simulink model "Test_openloop"  (R2017b)
settings: Solver=ode45  StartTime=0.0  StopTime=10  RelTol=1e-3
values from neighbouring files (symbols this model uses):
  Cdv = 0.02    [params.m]
  D = 0.55    [params.m]
  Ix = 1    [params.m]
  Ixy = 0.2    [params.m]
  Iy = 1    [params.m]
  Iz = 1    [params.m]
  Lx = b/2 + L_kr / sqrt(1 + tan(phi_kr1)^2 + tan(phi_kr1)^2)    [params.m]
  Ly = L_kr / sqrt(1 + tan(phi_kr1)^2 + tan(phi_kr1)^2) * tan(phi_kr2)    [params.m]
  Lz = a/2 + L_kr / sqrt(1 + tan(phi_kr1)^2 + tan(phi_kr1)^2) * tan(phi_kr1)    [params.m]
  M = [m 0 0 0 0 0 ... (first row only)    [params.m]
  m = 1    [params.m]
  rho = 1.22    [params.m]
  x_c = 0    [params.m]
  y_c = 0.005    [params.m]
settings Model: Creator=alexeimargun  LastModifiedBy=alexeimargun
settings DataIOCC: SaveFormat=StructureWithTime
settings OptimizationCC: LifeSpan=inf
settings DebuggingCC: SFExecutionAtInitializationDiag=none
settings HardwareCC: ProdBitPerSizeT=32  ProdBitPerPtrDiffT=32  ProdWordSize=32  ProdHWDeviceType=Specified
settings CodeAppCC: StateflowObjectComments=on
settings GRTTargetCC: GeneratePreprocessorConditionals=Disable all

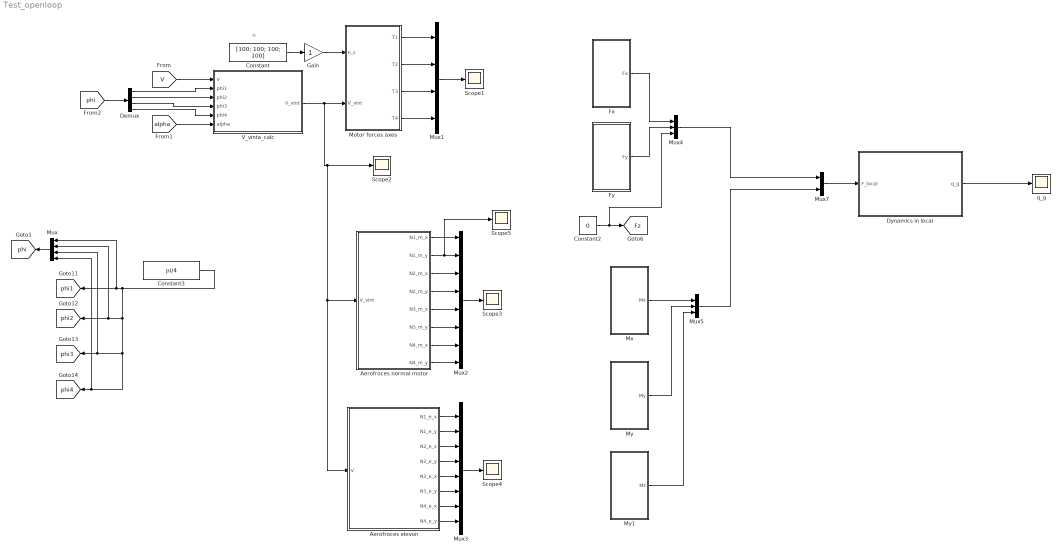
== system Test_openloop ==
  note: n
  Aerofroces elevon : Subsystem
  Aerofroces normal motor : Subsystem
  Constant : Constant  Value=[100; 100; 100; 100]
  Constant2 : Constant  Value=0
  Constant3 : Constant  Value=pi/4
  Demux : Demux
  Dynamics in local : Subsystem
  Fx : Subsystem
  Fy : Subsystem
  Gain : Gain
  Motor forces axes : Subsystem
  Mux : Mux
  Mux1 : Mux
  Mux2 : Mux  Inputs=8
  Mux3 : Mux  Inputs=8
  Mux4 : Mux  Inputs=3
  Mux5 : Mux  Inputs=3
  Mux7 : Mux  Inputs=2
  Mx : Subsystem
  My : Subsystem
  My1 : Subsystem
  Scope{1..5} (5 alike) : Scope
  V_vinta_calc : MATLAB Function  TreatAsAtomicUnit=on
  q_g : Scope
  tag scope: Fz=global, phi1=global, phi2=global, phi3=global, phi4=global, phi=global
  wires:
  Dynamics in local/1(q_g) -> q_g/1
  Motor forces axes/2(T2) -> Mux1/2
  Mux1/1 -> Scope1/1
  Motor forces axes/1(T1) -> Mux1/1
  Constant/1 -> Gain/1
  Motor forces axes/3(T3) -> Mux1/3
  Motor forces axes/4(T4) -> Mux1/4
  [V] -> V_vinta_calc/1(V)
  [alpha] -> V_vinta_calc/6(alpha)
  Gain/1 -> Motor forces axes/1(n_s)
  V_vinta_calc/1(V_vint) -> Aerofroces elevon/1(V), Aerofroces normal motor/1(V_vint), Scope2/1, Motor forces axes/2(V_vint)
  Aerofroces elevon/7(N4_e_x) -> Mux3/7
  Aerofroces elevon/3(N2_e_x) -> Mux3/3
  Aerofroces normal motor/4(N2_m_y) -> Mux2/4
  Aerofroces normal motor/7(N4_m_x) -> Mux2/7
  Aerofroces normal motor/5(N3_m_x) -> Mux2/5
  Aerofroces elevon/2(N1_e_y) -> Mux3/2
  Mux3/1 -> Scope4/1
  Aerofroces elevon/5(N3_e_x) -> Mux3/5
  Aerofroces normal motor/8(N4_m_y) -> Mux2/8
  Mux2/1 -> Scope3/1
  Aerofroces elevon/1(N1_e_x) -> Mux3/1
  Aerofroces normal motor/3(N2_m_x) -> Mux2/3
  Aerofroces elevon/6(N3_e_y) -> Mux3/6
  Aerofroces normal motor/6(N3_m_y) -> Mux2/6
  Aerofroces elevon/4(N2_e_y) -> Mux3/4
  Aerofroces elevon/8(N4_e_y) -> Mux3/8
  Aerofroces normal motor/2(N1_m_y) -> Scope5/1, Mux2/2
  Aerofroces normal motor/1(N1_m_x) -> Mux2/1
  Constant3/1 -> Mux/4, [phi4], Mux/3, [phi3], [phi2], Mux/2, [phi1], Mux/1
  Mux/1 -> [phi]
  [phi] -> Demux/1
  Demux/1 -> V_vinta_calc/2(phi1)
  Demux/2 -> V_vinta_calc/3(phi2)
  Demux/3 -> V_vinta_calc/4(phi3)
  Demux/4 -> V_vinta_calc/5(phi4)
  Constant2/1 -> Mux4/3, [Fz]
  Fy/1(Fy) -> Mux4/2
  Mux4/1 -> Mux7/1
  Mx/1(Mx) -> Mux5/1
  My/1(My) -> Mux5/2
  My1/1(Mz) -> Mux5/3
  Mux5/1 -> Mux7/2
  Fx/1(Fx) -> Mux4/1
  Mux7/1 -> Dynamics in local/1(F_local)

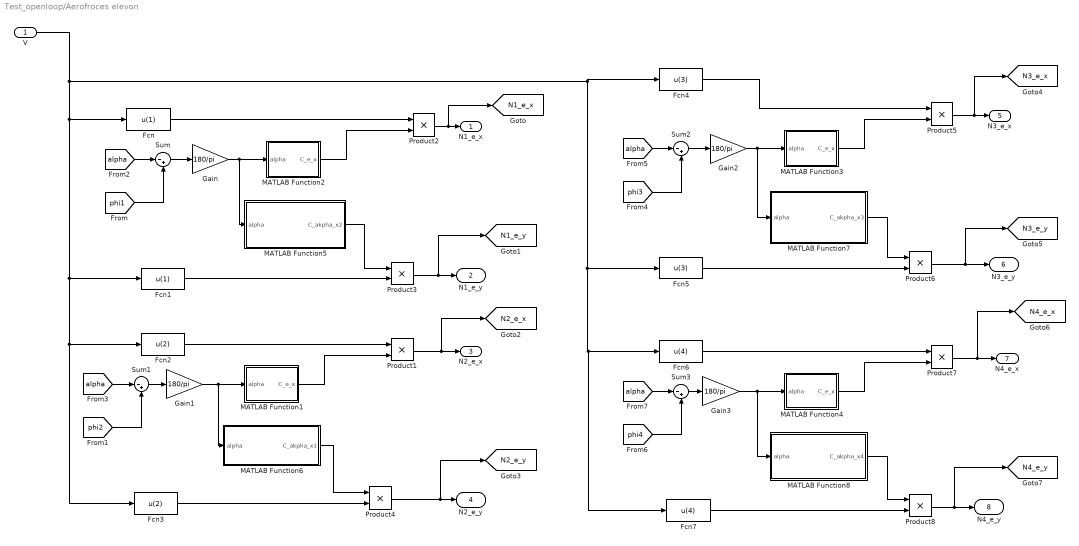
== system Test_openloop/Aerofroces elevon ==
  V : Inport
  Fcn : Fcn  Expr=u(1)
  Fcn1 : Fcn  Expr=u(1)
  Fcn2 : Fcn  Expr=u(2)
  Fcn3 : Fcn  Expr=u(2)
  Fcn4 : Fcn  Expr=u(3)
  Fcn5 : Fcn  Expr=u(3)
  Fcn6 : Fcn  Expr=u(4)
  Fcn7 : Fcn  Expr=u(4)
  Gain{,1..3} (4 alike) : Gain  Gain=180/pi
  MATLAB Function1 : MATLAB Function  TreatAsAtomicUnit=on
  MATLAB Function2 : MATLAB Function  TreatAsAtomicUnit=on
  MATLAB Function3 : MATLAB Function  TreatAsAtomicUnit=on
  MATLAB Function4 : MATLAB Function  TreatAsAtomicUnit=on
  MATLAB Function5 : MATLAB Function  TreatAsAtomicUnit=on
  MATLAB Function6 : MATLAB Function  TreatAsAtomicUnit=on
  MATLAB Function7 : MATLAB Function  TreatAsAtomicUnit=on
  MATLAB Function8 : MATLAB Function  TreatAsAtomicUnit=on
  Product{1..8} (8 alike) : Product
  Sum{,1..3} (4 alike) : Sum  Inputs=|-+
  N1_e_x : Outport
  N1_e_y : Outport  Port=2
  N2_e_x : Outport  Port=3
  N2_e_y : Outport  Port=4
  N3_e_x : Outport  Port=5
  N3_e_y : Outport  Port=6
  N4_e_x : Outport  Port=7
  N4_e_y : Outport  Port=8
  tag scope: N1_e_x=global, N1_e_y=global, N2_e_x=global, N2_e_y=global, N3_e_x=global, N3_e_y=global, N4_e_x=global, N4_e_y=global
  wires:
  Product3/1 -> [N1_e_y], N1_e_y/1
  Product2/1 -> [N1_e_x], N1_e_x/1
  Sum/1 -> Gain/1
  MATLAB Function5/1(C_akpha_x2) -> Product3/1
  MATLAB Function2/1(C_e_x) -> Product2/2
  [alpha] -> Sum1/1
  [phi2] -> Sum1/2
  V/1 -> Fcn7/1, Fcn6/1, Fcn5/1, Fcn4/1, Fcn2/1, Fcn3/1, Fcn1/1, Fcn/1
  MATLAB Function1/1(C_e_x) -> Product1/2
  MATLAB Function6/1(C_akpha_x1) -> Product4/1
  Sum1/1 -> Gain1/1
  Product1/1 -> [N2_e_x], N2_e_x/1
  Product4/1 -> [N2_e_y], N2_e_y/1
  Product6/1 -> [N3_e_y], N3_e_y/1
  Product5/1 -> [N3_e_x], N3_e_x/1
  Sum2/1 -> Gain2/1
  MATLAB Function7/1(C_akpha_x3) -> Product6/1
  MATLAB Function3/1(C_e_x) -> Product5/2
  [phi3] -> Sum2/2
  [alpha] -> Sum2/1
  [alpha] -> Sum3/1
  [phi4] -> Sum3/2
  MATLAB Function4/1(C_e_x) -> Product7/2
  MATLAB Function8/1(C_akpha_x4) -> Product8/1
  Sum3/1 -> Gain3/1
  Product7/1 -> [N4_e_x], N4_e_x/1
  Product8/1 -> [N4_e_y], N4_e_y/1
  Gain/1 -> MATLAB Function5/1(alpha), MATLAB Function2/1(alpha)
  Gain1/1 -> MATLAB Function6/1(alpha), MATLAB Function1/1(alpha)
  Gain2/1 -> MATLAB Function7/1(alpha), MATLAB Function3/1(alpha)
  Gain3/1 -> MATLAB Function8/1(alpha), MATLAB Function4/1(alpha)
  Fcn/1 -> Product2/1
  Fcn1/1 -> Product3/2
  Fcn2/1 -> Product1/1
  Fcn3/1 -> Product4/2
  Fcn4/1 -> Product5/1
  Fcn5/1 -> Product6/2
  Fcn6/1 -> Product7/1
  Fcn7/1 -> Product8/2
  [alpha] -> Sum/1
  [phi1] -> Sum/2

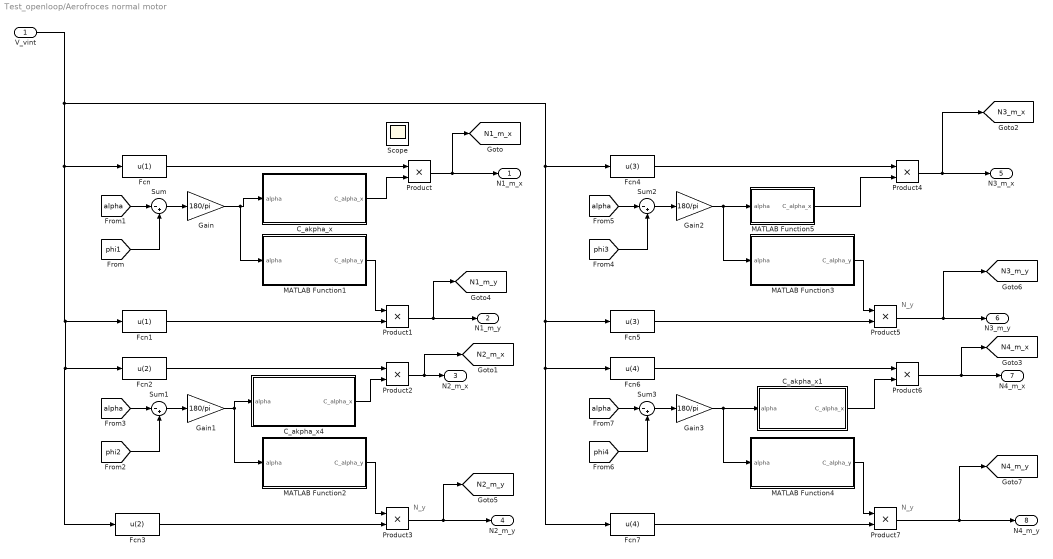
== system Test_openloop/Aerofroces normal motor ==
  note: N_y
  note: N_y
  note: N_y
  V_vint : Inport
  C_akpha_x : MATLAB Function  TreatAsAtomicUnit=on
  C_akpha_x1 : MATLAB Function  TreatAsAtomicUnit=on
  C_akpha_x4 : MATLAB Function  TreatAsAtomicUnit=on
  Fcn : Fcn  Expr=u(1)
  Fcn1 : Fcn  Expr=u(1)
  Fcn2 : Fcn  Expr=u(2)
  Fcn3 : Fcn  Expr=u(2)
  Fcn4 : Fcn  Expr=u(3)
  Fcn5 : Fcn  Expr=u(3)
  Fcn6 : Fcn  Expr=u(4)
  Fcn7 : Fcn  Expr=u(4)
  Gain{,1..3} (4 alike) : Gain  Gain=180/pi
  MATLAB Function1 : MATLAB Function  TreatAsAtomicUnit=on
  MATLAB Function2 : MATLAB Function  TreatAsAtomicUnit=on
  MATLAB Function3 : MATLAB Function  TreatAsAtomicUnit=on
  MATLAB Function4 : MATLAB Function  TreatAsAtomicUnit=on
  MATLAB Function5 : MATLAB Function  TreatAsAtomicUnit=on
  Product{,1..7} (8 alike) : Product
  Scope : Scope
  Sum{,1..3} (4 alike) : Sum  Inputs=|-+
  N1_m_x : Outport
  N1_m_y : Outport  Port=2
  N2_m_x : Outport  Port=3
  N2_m_y : Outport  Port=4
  N3_m_x : Outport  Port=5
  N3_m_y : Outport  Port=6
  N4_m_x : Outport  Port=7
  N4_m_y : Outport  Port=8
  tag scope: N1_m_x=global, N1_m_y=global, N2_m_x=global, N2_m_y=global, N3_m_x=global, N3_m_y=global, N4_m_x=global, N4_m_y=global
  wires:
  Product1/1 -> [N1_m_y], N1_m_y/1
  C_akpha_x/1(C_alpha_x) -> Product/2
  MATLAB Function1/1(C_alpha_y) -> Product1/1
  [alpha] -> Sum/1
  Sum/1 -> Gain/1
  [phi1] -> Sum/2
  Gain1/1 -> MATLAB Function2/1(alpha), C_akpha_x4/1(alpha)
  [phi2] -> Sum1/2
  Sum1/1 -> Gain1/1
  [alpha] -> Sum1/1
  MATLAB Function2/1(C_alpha_y) -> Product3/1
  C_akpha_x4/1(C_alpha_x) -> Product2/2
  Product2/1 -> [N2_m_x], N2_m_x/1
  Product3/1 -> [N2_m_y], N2_m_y/1
  Product7/1 -> [N4_m_y], N4_m_y/1
  Product6/1 -> [N4_m_x], N4_m_x/1
  V_vint/1 -> Fcn5/1, Fcn6/1, Fcn7/1, Fcn4/1, Fcn/1, Fcn3/1, Fcn2/1, Fcn1/1
  C_akpha_x1/1(C_alpha_x) -> Product6/2
  MATLAB Function4/1(C_alpha_y) -> Product7/1
  [alpha] -> Sum3/1
  Sum3/1 -> Gain3/1
  [phi4] -> Sum3/2
  Gain3/1 -> MATLAB Function4/1(alpha), C_akpha_x1/1(alpha)
  Gain2/1 -> MATLAB Function3/1(alpha), MATLAB Function5/1(alpha)
  [phi3] -> Sum2/2
  Sum2/1 -> Gain2/1
  [alpha] -> Sum2/1
  MATLAB Function3/1(C_alpha_y) -> Product5/1
  MATLAB Function5/1(C_alpha_x) -> Product4/2
  Product4/1 -> [N3_m_x], N3_m_x/1
  Product5/1 -> [N3_m_y], N3_m_y/1
  Product/1 -> [N1_m_x], N1_m_x/1
  Gain/1 -> MATLAB Function1/1(alpha), C_akpha_x/1(alpha)
  Fcn/1 -> Product/1
  Fcn1/1 -> Product1/2
  Fcn2/1 -> Product2/1
  Fcn3/1 -> Product3/2
  Fcn4/1 -> Product4/1
  Fcn5/1 -> Product5/2
  Fcn6/1 -> Product6/1
  Fcn7/1 -> Product7/2

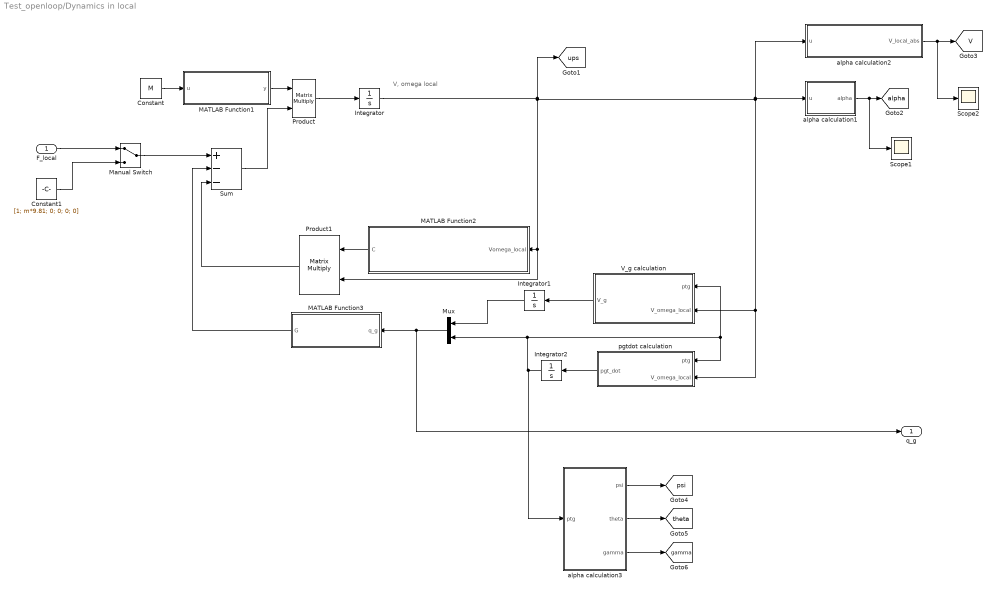
== system Test_openloop/Dynamics in local ==
  note: V, omega local
  F_local : Inport
  Constant : Constant  Value=M
  Constant1 : Constant  Value=[1; m*9.81; 0; 0; 0; 0]
  Integrator : Integrator
  Integrator1 : Integrator  InitialCondition=[0;0;0]
  Integrator2 : Integrator  InitialCondition=[0;0;0]
  MATLAB Function1 : MATLAB Function  TreatAsAtomicUnit=on
  MATLAB Function2 : MATLAB Function  TreatAsAtomicUnit=on
  MATLAB Function3 : MATLAB Function  TreatAsAtomicUnit=on
  Manual Switch : ManualSwitch
  Mux : Mux  Inputs=2
  Product : Product  Multiplication=Matrix(*)
  Product1 : Product  Multiplication=Matrix(*)
  Scope1 : Scope
  Scope2 : Scope
  Sum : Sum  Inputs=+--
  V_g calculation : MATLAB Function  TreatAsAtomicUnit=on
  alpha calculation1 : MATLAB Function  TreatAsAtomicUnit=on
  alpha calculation2 : MATLAB Function  TreatAsAtomicUnit=on
  alpha calculation3 : MATLAB Function  TreatAsAtomicUnit=on
  pgtdot calculation : MATLAB Function  TreatAsAtomicUnit=on
  q_g : Outport
  tag scope: V=global, alpha=global, gamma=global, psi=global, theta=global, ups=global
  wires:
  MATLAB Function1/1(y) -> Product/1
  Product1/1 -> Sum/3
  Integrator2/1 -> alpha calculation3/1(ptg), V_g calculation/1(ptg), pgtdot calculation/1(ptg), Mux/2
  Integrator/1 -> Product1/2, MATLAB Function2/1(Vomega_local), alpha calculation2/1(u), alpha calculation1/1(u), V_g calculation/2(V_omega_local), pgtdot calculation/2(V_omega_local), [ups]
  Mux/1 -> q_g/1, MATLAB Function3/1(q_g)
  pgtdot calculation/1(pgt_dot) -> Integrator2/1
  MATLAB Function3/1(G) -> Sum/2
  Sum/1 -> Product/2
  Integrator1/1 -> Mux/1
  Constant/1 -> MATLAB Function1/1(u)
  MATLAB Function2/1(C) -> Product1/1
  Product/1 -> Integrator/1
  V_g calculation/1(V_g) -> Integrator1/1
  alpha calculation1/1(alpha) -> Scope1/1, [alpha]
  alpha calculation2/1(V_local_abs) -> Scope2/1, [V]
  Constant1/1 -> Manual Switch/2
  Manual Switch/1 -> Sum/1
  F_local/1 -> Manual Switch/1
  alpha calculation3/1(psi) -> [psi]
  alpha calculation3/2(theta) -> [theta]
  alpha calculation3/3(gamma) -> [gamma]

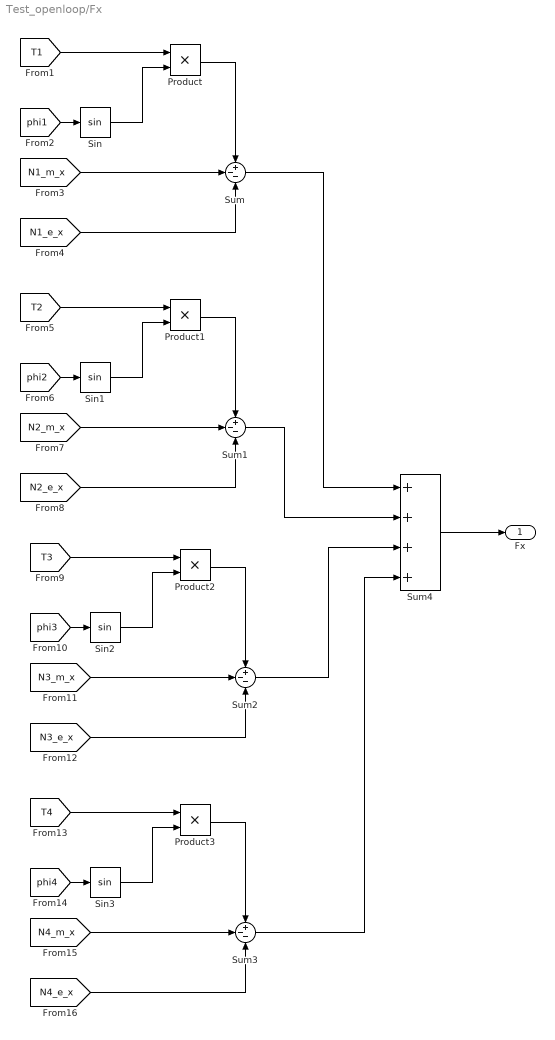
== system Test_openloop/Fx ==
  Product{,1..3} (4 alike) : Product
  Sin{,1..3} (4 alike) : Trigonometry
  Sum{,1..3} (4 alike) : Sum  Inputs=+--
  Sum4 : Sum  Inputs=++++
  Fx : Outport
  wires:
  [phi3] -> Sin2/1
  Product2/1 -> Sum2/1
  Sin2/1 -> Product2/2
  [phi4] -> Sin3/1
  [N3_e_x] -> Sum2/3
  [T1] -> Product/1
  Product/1 -> Sum/1
  [T2] -> Product1/1
  Sin1/1 -> Product1/2
  [N2_m_x] -> Sum1/2
  Product3/1 -> Sum3/1
  Sum/1 -> Sum4/1
  [phi2] -> Sin1/1
  [N1_m_x] -> Sum/2
  [N1_e_x] -> Sum/3
  [T3] -> Product2/1
  Sin3/1 -> Product3/2
  Sin/1 -> Product/2
  [N4_m_x] -> Sum3/2
  [N3_m_x] -> Sum2/2
  [phi1] -> Sin/1
  [T4] -> Product3/1
  Sum2/1 -> Sum4/3
  Sum1/1 -> Sum4/2
  [N4_e_x] -> Sum3/3
  Product1/1 -> Sum1/1
  Sum3/1 -> Sum4/4
  [N2_e_x] -> Sum1/3
  Sum4/1 -> Fx/1

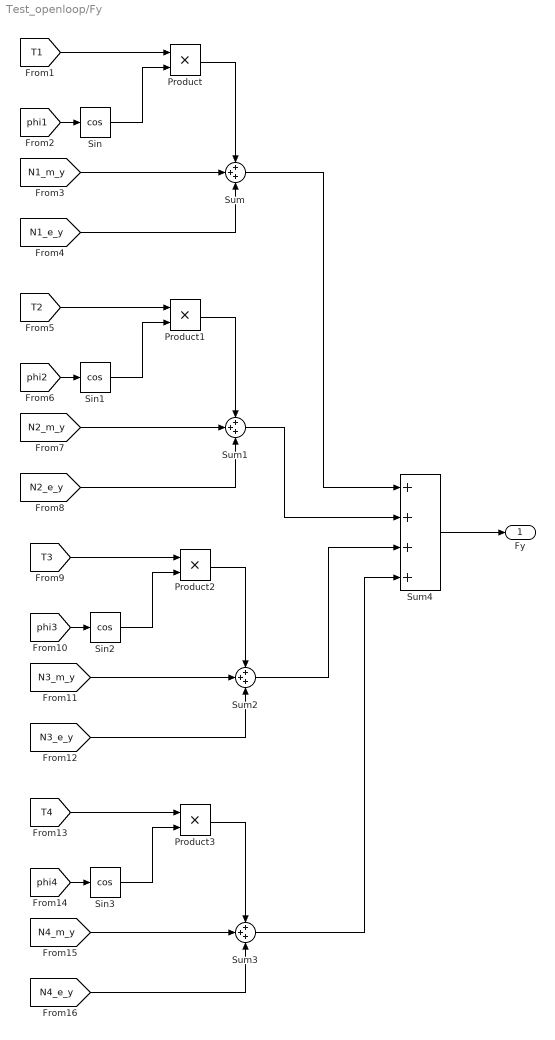
== system Test_openloop/Fy ==
  Product{,1..3} (4 alike) : Product
  Sin{,1..3} (4 alike) : Trigonometry  Operator=cos
  Sum{,1..3} (4 alike) : Sum  Inputs=+++
  Sum4 : Sum  Inputs=++++
  Fy : Outport
  wires:
  Sum4/1 -> Fy/1
  [N2_e_y] -> Sum1/3
  Sum3/1 -> Sum4/4
  Product1/1 -> Sum1/1
  [N4_e_y] -> Sum3/3
  Sum1/1 -> Sum4/2
  Sum2/1 -> Sum4/3
  [T4] -> Product3/1
  [phi1] -> Sin/1
  [N3_m_y] -> Sum2/2
  [N4_m_y] -> Sum3/2
  Sin/1 -> Product/2
  Sin3/1 -> Product3/2
  [T3] -> Product2/1
  [N1_e_y] -> Sum/3
  [N1_m_y] -> Sum/2
  [phi2] -> Sin1/1
  Sum/1 -> Sum4/1
  Product3/1 -> Sum3/1
  [N2_m_y] -> Sum1/2
  Sin1/1 -> Product1/2
  [T2] -> Product1/1
  Product/1 -> Sum/1
  [T1] -> Product/1
  [N3_e_y] -> Sum2/3
  [phi4] -> Sin3/1
  Sin2/1 -> Product2/2
  Product2/1 -> Sum2/1
  [phi3] -> Sin2/1

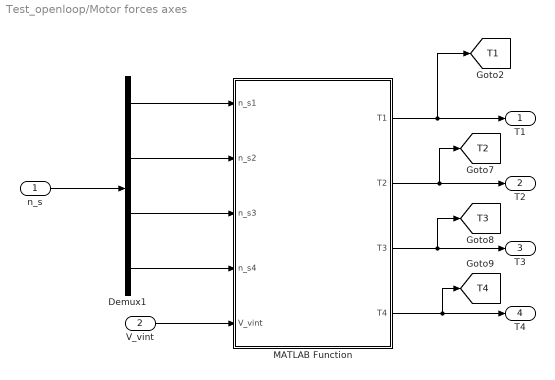
== system Test_openloop/Motor forces axes ==
  n_s : Inport
  V_vint : Inport  Port=2
  Demux1 : Demux
  MATLAB Function : MATLAB Function  TreatAsAtomicUnit=on
  T1 : Outport
  T2 : Outport  Port=2
  T3 : Outport  Port=3
  T4 : Outport  Port=4
  tag scope: T1=global, T2=global, T3=global, T4=global
  wires:
  MATLAB Function/3(T3) -> [T3], T3/1
  MATLAB Function/4(T4) -> [T4], T4/1
  Demux1/1 -> MATLAB Function/1(n_s1)
  Demux1/3 -> MATLAB Function/3(n_s3)
  Demux1/4 -> MATLAB Function/4(n_s4)
  V_vint/1 -> MATLAB Function/5(V_vint)
  MATLAB Function/2(T2) -> [T2], T2/1
  Demux1/2 -> MATLAB Function/2(n_s2)
  MATLAB Function/1(T1) -> [T1], T1/1
  n_s/1 -> Demux1/1

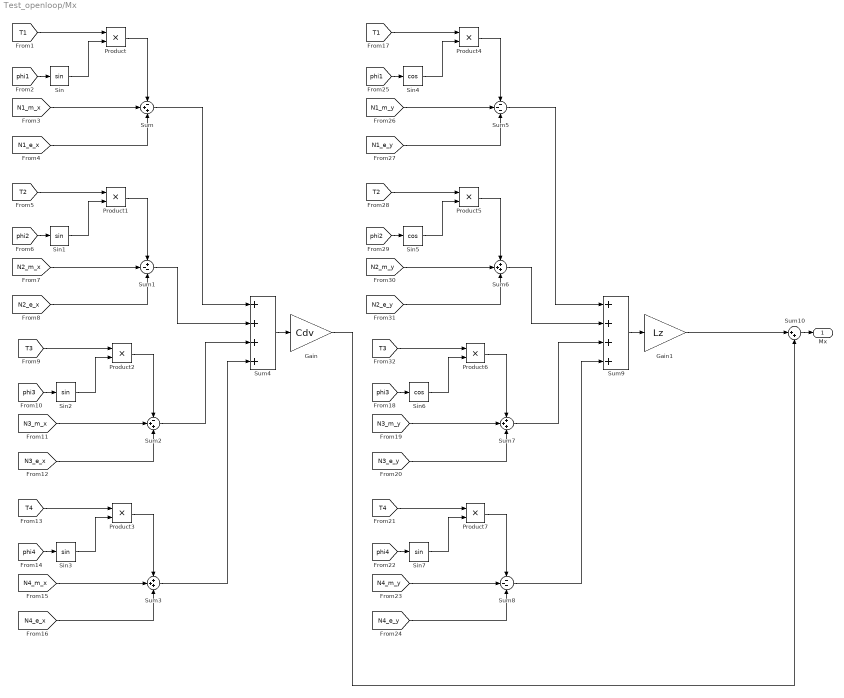
== system Test_openloop/Mx ==
  Gain : Gain  Gain=Cdv
  Gain1 : Gain  Gain=Lz
  Product{,1..7} (8 alike) : Product
  Sin{,1..3,7} (5 alike) : Trigonometry
  Sin4 : Trigonometry  Operator=cos
  Sin5 : Trigonometry  Operator=cos
  Sin6 : Trigonometry  Operator=cos
  Sum : Sum  Inputs=-++
  Sum1 : Sum  Inputs=+--
  Sum10 : Sum  Inputs=|++
  Sum2 : Sum  Inputs=-++
  Sum3 : Sum  Inputs=+++
  Sum4 : Sum  Inputs=++++
  Sum5 : Sum  Inputs=---
  Sum6 : Sum  Inputs=+++
  Sum7 : Sum  Inputs=+++
  Sum8 : Sum  Inputs=---
  Sum9 : Sum  Inputs=++++
  Mx : Outport
  wires:
  [N2_e_x] -> Sum1/3
  [phi3] -> Sin6/1
  Sum3/1 -> Sum4/4
  Product1/1 -> Sum1/1
  [N4_e_x] -> Sum3/3
  Sum8/1 -> Sum9/4
  Sum1/1 -> Sum4/2
  [N4_e_y] -> Sum8/3
  [T1] -> Product4/1
  Sin6/1 -> Product6/2
  Sum9/1 -> Gain1/1
  Product7/1 -> Sum8/1
  Sum5/1 -> Sum9/1
  Sum2/1 -> Sum4/3
  [T4] -> Product3/1
  [phi1] -> Sin/1
  Sum7/1 -> Sum9/3
  Product6/1 -> Sum7/1
  Sum6/1 -> Sum9/2
  [N3_e_y] -> Sum7/3
  [T3] -> Product6/1
  [N3_m_x] -> Sum2/2
  [phi1] -> Sin4/1
  [N4_m_x] -> Sum3/2
  Sin/1 -> Product/2
  Sin3/1 -> Product3/2
  Product4/1 -> Sum5/1
  [T3] -> Product2/1
  [phi2] -> Sin5/1
  Sin4/1 -> Product4/2
  Sum4/1 -> Gain/1
  [N1_e_x] -> Sum/3
  [N1_m_x] -> Sum/2
  [T2] -> Product5/1
  Sin7/1 -> Product7/2
  [phi2] -> Sin1/1
  [N1_e_y] -> Sum5/3
  Sum/1 -> Sum4/1
  [phi4] -> Sin7/1
  [T4] -> Product7/1
  Product3/1 -> Sum3/1
  Product5/1 -> Sum6/1
  [N2_m_x] -> Sum1/2
  Sin5/1 -> Product5/2
  Sin1/1 -> Product1/2
  Gain1/1 -> Sum10/1
  [N2_e_y] -> Sum6/3
  [N2_m_y] -> Sum6/2
  [N1_m_y] -> Sum5/2
  [T2] -> Product1/1
  Product/1 -> Sum/1
  [N3_m_y] -> Sum7/2
  [T1] -> Product/1
  [N3_e_x] -> Sum2/3
  [N4_m_y] -> Sum8/2
  Gain/1 -> Sum10/2
  Sum10/1 -> Mx/1
  [phi4] -> Sin3/1
  Sin2/1 -> Product2/2
  Product2/1 -> Sum2/1
  [phi3] -> Sin2/1

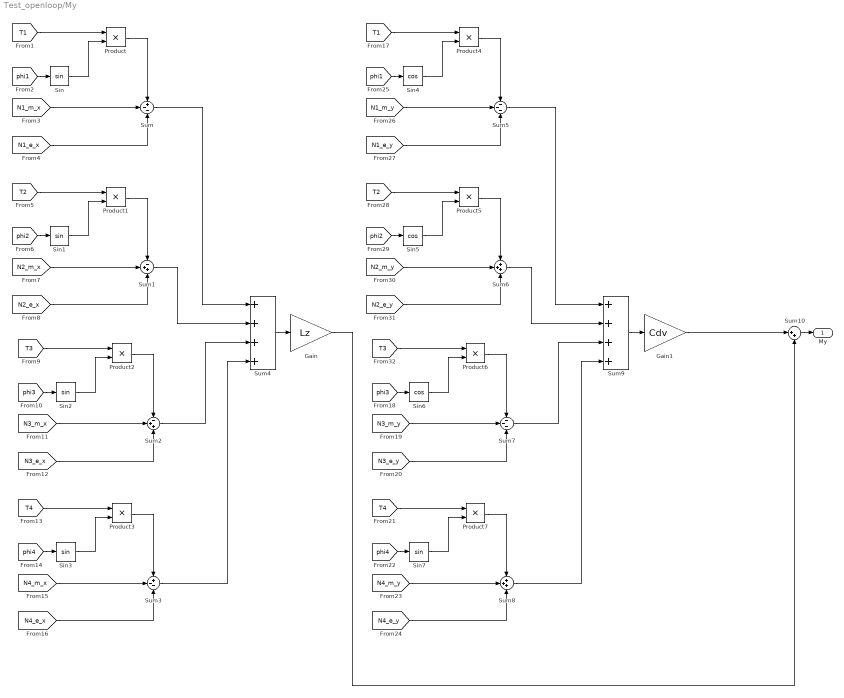
== system Test_openloop/My ==
  Gain : Gain  Gain=Lz
  Gain1 : Gain  Gain=Cdv
  Product{,1..7} (8 alike) : Product
  Sin{,1..3,7} (5 alike) : Trigonometry
  Sin4 : Trigonometry  Operator=cos
  Sin5 : Trigonometry  Operator=cos
  Sin6 : Trigonometry  Operator=cos
  Sum : Sum  Inputs=+--
  Sum1 : Sum  Inputs=-++
  Sum10 : Sum  Inputs=|++
  Sum2 : Sum  Inputs=-++
  Sum3 : Sum  Inputs=+--
  Sum4 : Sum  Inputs=++++
  Sum5 : Sum  Inputs=---
  Sum6 : Sum  Inputs=+++
  Sum7 : Sum  Inputs=---
  Sum8 : Sum  Inputs=+++
  Sum9 : Sum  Inputs=++++
  My : Outport
  wires:
  [phi3] -> Sin2/1
  Product2/1 -> Sum2/1
  Sin2/1 -> Product2/2
  [phi4] -> Sin3/1
  Sum10/1 -> My/1
  Gain/1 -> Sum10/2
  [N4_m_y] -> Sum8/2
  [N3_e_x] -> Sum2/3
  [T1] -> Product/1
  [N3_m_y] -> Sum7/2
  Product/1 -> Sum/1
  [T2] -> Product1/1
  [N1_m_y] -> Sum5/2
  [N2_m_y] -> Sum6/2
  [N2_e_y] -> Sum6/3
  Gain1/1 -> Sum10/1
  Sin1/1 -> Product1/2
  Sin5/1 -> Product5/2
  [N2_m_x] -> Sum1/2
  Product5/1 -> Sum6/1
  Product3/1 -> Sum3/1
  [T4] -> Product7/1
  [phi4] -> Sin7/1
  Sum/1 -> Sum4/1
  [N1_e_y] -> Sum5/3
  [phi2] -> Sin1/1
  Sin7/1 -> Product7/2
  [T2] -> Product5/1
  [N1_m_x] -> Sum/2
  [N1_e_x] -> Sum/3
  Sum4/1 -> Gain/1
  Sin4/1 -> Product4/2
  [phi2] -> Sin5/1
  [T3] -> Product2/1
  Product4/1 -> Sum5/1
  Sin3/1 -> Product3/2
  Sin/1 -> Product/2
  [N4_m_x] -> Sum3/2
  [phi1] -> Sin4/1
  [N3_m_x] -> Sum2/2
  [T3] -> Product6/1
  [N3_e_y] -> Sum7/3
  Sum6/1 -> Sum9/2
  Product6/1 -> Sum7/1
  Sum7/1 -> Sum9/3
  [phi1] -> Sin/1
  [T4] -> Product3/1
  Sum2/1 -> Sum4/3
  Sum5/1 -> Sum9/1
  Product7/1 -> Sum8/1
  Sum9/1 -> Gain1/1
  Sin6/1 -> Product6/2
  [T1] -> Product4/1
  [N4_e_y] -> Sum8/3
  Sum1/1 -> Sum4/2
  Sum8/1 -> Sum9/4
  [N4_e_x] -> Sum3/3
  Product1/1 -> Sum1/1
  Sum3/1 -> Sum4/4
  [phi3] -> Sin6/1
  [N2_e_x] -> Sum1/3

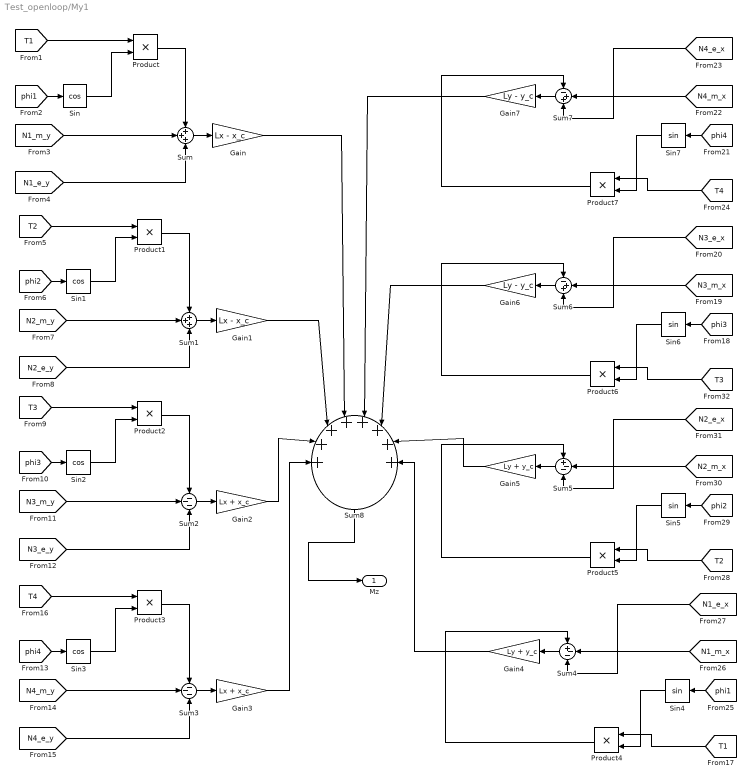
== system Test_openloop/My1 ==
  Gain : Gain  Gain=Lx - x_c
  Gain1 : Gain  Gain=Lx - x_c
  Gain2 : Gain  Gain=Lx + x_c
  Gain3 : Gain  Gain=Lx + x_c
  Gain4 : Gain  Gain=Ly + y_c
  Gain5 : Gain  Gain=Ly + y_c
  Gain6 : Gain  Gain=Ly - y_c
  Gain7 : Gain  Gain=Ly - y_c
  Product{,1..7} (8 alike) : Product
  Sin{,1..3} (4 alike) : Trigonometry  Operator=cos
  Sin{4..7} (4 alike) : Trigonometry
  Sum : Sum  Inputs=+++
  Sum1 : Sum  Inputs=+++
  Sum2 : Sum  Inputs=---
  Sum3 : Sum  Inputs=---
  Sum4 : Sum  Inputs=+--
  Sum5 : Sum  Inputs=+--
  Sum6 : Sum  Inputs=-++
  Sum7 : Sum  Inputs=-++
  Sum8 : Sum  Inputs=++++++++
  Mz : Outport
  wires:
  [phi1] -> Sin/1
  Sin/1 -> Product/2
  [N1_e_y] -> Sum/3
  [N1_m_y] -> Sum/2
  Product/1 -> Sum/1
  [T1] -> Product/1
  Sum/1 -> Gain/1
  Sum1/1 -> Gain1/1
  [T2] -> Product1/1
  Product1/1 -> Sum1/1
  [N2_m_y] -> Sum1/2
  [N2_e_y] -> Sum1/3
  Sin1/1 -> Product1/2
  [phi2] -> Sin1/1
  [phi3] -> Sin2/1
  Sin2/1 -> Product2/2
  [N3_e_y] -> Sum2/3
  [N3_m_y] -> Sum2/2
  Product2/1 -> Sum2/1
  [T3] -> Product2/1
  Sum2/1 -> Gain2/1
  Sum3/1 -> Gain3/1
  [T4] -> Product3/1
  Product3/1 -> Sum3/1
  [N4_m_y] -> Sum3/2
  [N4_e_y] -> Sum3/3
  Sin3/1 -> Product3/2
  [phi4] -> Sin3/1
  [phi4] -> Sin7/1
  Sin7/1 -> Product7/2
  [N4_e_x] -> Sum7/3
  [N4_m_x] -> Sum7/2
  Product7/1 -> Sum7/1
  [T4] -> Product7/1
  Sum7/1 -> Gain7/1
  Sum6/1 -> Gain6/1
  [T3] -> Product6/1
  Product6/1 -> Sum6/1
  [N3_m_x] -> Sum6/2
  [N3_e_x] -> Sum6/3
  Sin6/1 -> Product6/2
  [phi3] -> Sin6/1
  [phi2] -> Sin5/1
  Sin5/1 -> Product5/2
  [N2_e_x] -> Sum5/3
  [N2_m_x] -> Sum5/2
  Product5/1 -> Sum5/1
  [T2] -> Product5/1
  Sum5/1 -> Gain5/1
  Sum4/1 -> Gain4/1
  [T1] -> Product4/1
  Product4/1 -> Sum4/1
  [N1_m_x] -> Sum4/2
  [N1_e_x] -> Sum4/3
  Sin4/1 -> Product4/2
  [phi1] -> Sin4/1
  Gain3/1 -> Sum8/1
  Gain4/1 -> Sum8/8
  Gain5/1 -> Sum8/7
  Gain2/1 -> Sum8/2
  Gain1/1 -> Sum8/3
  Gain6/1 -> Sum8/6
  Gain/1 -> Sum8/4
  Gain7/1 -> Sum8/5
  Sum8/1 -> Mz/1

== matlab function Test_openloop/Dynamics in local/MATLAB Function1 ==
  data: u input; y output
function y = inversion_matrix(u)

y = inv(u);

== matlab function Test_openloop/Dynamics in local/alpha calculation1 ==
  data: u input; alpha output
function alpha = fcn(u)
V = u(1:3);
if V(1) == 0
    alpha = pi/2;
else
    alpha = atan(V(2)/V(1));
end;

== matlab function Test_openloop/Dynamics in local/MATLAB Function2 ==
  data: Vomega_local input; C output; Ix parameter; Iy parameter; Iz parameter; Ixy parameter; m parameter
function C = C_calculation(Vomega_local, Ix, Iy, Iz, Ixy, m)
omega_x = Vomega_local(4);
omega_y = Vomega_local(5);
omega_z = Vomega_local(6);

c12 = -m * omega_z;
c13 = m * omega_y;
c21 = m * omega_z;
c23 = -m* omega_x;
c31 = -m*omega_y;
c32 = m*omega_x;
c46 = (Iz-Iy)*omega_y + Ixy *omega_x;
c56 = (Ix - Iz)*omega_x - Ixy*omega_y;
c64 = -Ixy * omega_x;
c65 = (Iy-Ix)*omega_x + Ixy * omega_y;


C = [0 c12 c13 0 0 0;
     c21 0 c23 0 0 0;
     c31 c32 0 0 0 0;
     0 0 0 0 0 c46;
     0 0 0 0 0 c56;
     0 0 0 c64 c65 0];

== matlab function Test_openloop/Dynamics in local/MATLAB Function3 ==
  data: q_g input; G output; m parameter
function G = G_calculation(q_g, m)
theta = q_g(5);
gamma = q_g(6);
G = [m*9.81*sin(theta);
     m*9.81*cos(theta)*cos(gamma);
     -m*9.81*cos(theta)*sin(gamma);
      0;
      0;
      0];

== matlab function Test_openloop/Motor forces axes/MATLAB Function ==
  data: T1 output; n_s1 input; n_s2 input; n_s3 input; n_s4 input; V_vint input; rho parameter; D parameter; T2 output; T3 output; T4 output
function [T1, T2, T3, T4] = Force_T(n_s1, n_s2, n_s3, n_s4, V_vint, rho, D)

J1 = V_vint(1) / n_s1 / D;
J2 = V_vint(2) / n_s2 / D;
J3 = V_vint(3) / n_s3 / D;
J4 = V_vint(4) / n_s4 / D;

c_t1 = -0.1903 * (J1^2) - 0.0423 * J1 + 0.0959;
c_t2 = -0.1903 * (J2^2) - 0.0423 * J2 + 0.0959;
c_t3 = -0.1903 * (J3^2) - 0.0423 * J3 + 0.0959;
c_t4 = -0.1903 * (J4^2) - 0.0423 * J4 + 0.0959;

T1 = rho * c_t1 * (n_s1^2) * (D^4);
T2 = rho * c_t2 * (n_s2^2) * (D^4);
T3 = rho * c_t3 * (n_s3^2) * (D^4);
T4 = rho * c_t4 * (n_s4^2) * (D^4);

== matlab function Test_openloop/Dynamics in local/pgtdot calculation ==
  data: ptg input; pgt_dot output; V_omega_local input
function pgt_dot = fcn(ptg, V_omega_local)

omega = V_omega_local(4:6);

psi_dot = (omega(2)*cos(ptg(3))-omega(3)*sin(ptg(3)))/cos(ptg(2));
theta_dot = omega(2)*sin(ptg(3))+omega(3)*cos(ptg(3));
gamma_dot = omega(1)-tan(ptg(2))*(omega(2)*cos(ptg(3))-omega(3)*sin(ptg(3)));

pgt_dot = [psi_dot; theta_dot; gamma_dot];

== matlab function Test_openloop/Dynamics in local/V_g calculation ==
  data: ptg input; V_g output; V_omega_local input
function V_g = fcn(ptg, V_omega_local)

V = V_omega_local(1:3);

Gamma1 = [cos(ptg(1))*cos(ptg(2)) sin(ptg(2)) -sin(ptg(1))*cos(ptg(2));
    -cos(ptg(1))*sin(ptg(2))*cos(ptg(3))+sin(ptg(1))*sin(ptg(3)) cos(ptg(2))*cos(ptg(3)) cos(ptg(1))*sin(ptg(3))+sin(ptg(1))*sin(ptg(2))*cos(ptg(3));
    cos(ptg(1))*sin(ptg(2))*sin(ptg(3))+sin(ptg(1))*cos(ptg(3)) -cos(ptg(2))*sin(ptg(3)) cos(ptg(1))*cos(ptg(3))-sin(ptg(1))*sin(ptg(2))*sin(ptg(3))];

V_g=Gamma1'*V;

== matlab function Test_openloop/Dynamics in local/alpha calculation2 ==
  data: u input; V_local_abs output
function V_local_abs = fcn(u)
V = u(1:3);
V_local_abs = sqrt(V(1)^2 + V(2)^2 + V(3)^2);

== matlab function Test_openloop/V_vinta_calc ==
  data: V input; V_vint output; phi1 input; phi2 input; phi3 input; phi4 input; alpha input
function V_vint = fcn(V, phi1, phi2, phi3, phi4, alpha)

V_vint1 = V*cos(alpha)*cos(phi1);
V_vint2 = V*cos(alpha)*cos(phi2);
V_vint3 = V*cos(alpha)*cos(phi3);
V_vint4 = V*cos(alpha)*cos(phi4);

V_vint=[V_vint1; V_vint2; V_vint3; V_vint4];

== matlab function Test_openloop/Aerofroces elevon/MATLAB Function1 ==
  data: alpha input; C_e_x output
function C_e_x = fcn(alpha)
if alpha <30
    C_e_x = 0.000014*alpha^2 +0.000376*alpha + 0.002834;
else
     C_e_x = -0.000009*alpha^2 +0.001686*alpha - 0.014520;
end

== matlab function Test_openloop/Aerofroces normal motor/MATLAB Function1 ==
  data: alpha input; C_alpha_y output
function C_alpha_y = fcn(alpha)
if alpha <4
    C_alpha_y = 0.0714*alpha + 0.7908;
else
    C_alpha_y = -0.000643*alpha^2 + 0.066781*alpha + 0.816948;
end

== matlab function Test_openloop/Aerofroces normal motor/MATLAB Function2 ==
  data: alpha input; C_alpha_y output
function C_alpha_y = fcn(alpha)
if alpha <4
    C_alpha_y = 0.0714*alpha + 0.7908;
else
    C_alpha_y = -0.000643*alpha^2 + 0.066781*alpha + 0.816948;
end

== matlab function Test_openloop/Aerofroces elevon/MATLAB Function3 ==
  data: alpha input; C_e_x output
function C_e_x = fcn(alpha)
if alpha <30
    C_e_x = 0.000014*alpha^2 +0.000376*alpha + 0.002834;
else
     C_e_x = -0.000009*alpha^2 +0.001686*alpha - 0.014520;
end

== matlab function Test_openloop/Aerofroces elevon/MATLAB Function2 ==
  data: alpha input; C_e_x output
function C_e_x = fcn(alpha)
if alpha <30
    C_e_x = 0.000014*alpha^2 +0.000376*alpha + 0.002834;
else
     C_e_x = -0.000009*alpha^2 +0.001686*alpha - 0.014520;
end

== matlab function Test_openloop/Aerofroces elevon/MATLAB Function4 ==
  data: alpha input; C_e_x output
function C_e_x = fcn(alpha)
if alpha <30
    C_e_x = 0.000014*alpha^2 +0.000376*alpha + 0.002834;
else
     C_e_x = -0.000009*alpha^2 +0.001686*alpha - 0.014520;
end

== matlab function Test_openloop/Aerofroces normal motor/MATLAB Function3 ==
  data: alpha input; C_alpha_y output
function C_alpha_y = fcn(alpha)
if alpha <4
    C_alpha_y = 0.0714*alpha + 0.7908;
else
    C_alpha_y = -0.000643*alpha^2 + 0.066781*alpha + 0.816948;
end

== matlab function Test_openloop/Aerofroces normal motor/C_akpha_x ==
  data: alpha input; C_alpha_x output
function C_alpha_x = fcn(alpha)
C_alpha_x = 0.000455*alpha^2+0.009337*alpha+0.068991;

== matlab function Test_openloop/Aerofroces normal motor/C_akpha_x4 ==
  data: alpha input; C_alpha_x output
function C_alpha_x = fcn(alpha)
C_alpha_x = 0.000455 * alpha^2 +0.009337* alpha + 0.068991;

== matlab function Test_openloop/Aerofroces normal motor/MATLAB Function4 ==
  data: alpha input; C_alpha_y output
function C_alpha_y = fcn(alpha)
if alpha <4
    C_alpha_y = 0.0714*alpha + 0.7908;
else
    C_alpha_y = -0.000643*alpha^2 + 0.066781*alpha + 0.816948;
end

== matlab function Test_openloop/Aerofroces normal motor/C_akpha_x1 ==
  data: alpha input; C_alpha_x output
function C_alpha_x = fcn(alpha)
C_alpha_x = 0.000455 * alpha^2 +0.009337* alpha + 0.068991;

== matlab function Test_openloop/Aerofroces elevon/MATLAB Function5 ==
  data: alpha input; C_akpha_x2 output
function C_akpha_x2 = fcn(alpha)
C_akpha_x2 = 0.00000019*alpha^3 - 0.00004332*alpha^2+0.00233089*alpha;

== matlab function Test_openloop/Aerofroces elevon/MATLAB Function6 ==
  data: alpha input; C_akpha_x1 output
function C_akpha_x1 = fcn(alpha)
C_akpha_x1 = 0.00000019*alpha^3 - 0.00004332*alpha^2+0.00233089*alpha;

== matlab function Test_openloop/Aerofroces elevon/MATLAB Function7 ==
  data: alpha input; C_akpha_x3 output
function C_akpha_x3 = fcn(alpha)
C_akpha_x3 = 0.00000019*alpha^3 - 0.00004332*alpha^2+0.00233089*alpha;

== matlab function Test_openloop/Aerofroces elevon/MATLAB Function8 ==
  data: alpha input; C_akpha_x4 output
function C_akpha_x4 = fcn(alpha)
C_akpha_x4 = 0.00000019*alpha^3 - 0.00004332*alpha^2+0.00233089*alpha;

== matlab function Test_openloop/Aerofroces normal motor/MATLAB Function5 ==
  data: alpha input; C_alpha_x output
function C_alpha_x = fcn(alpha)
C_alpha_x = 0.000455 * alpha^2 +0.009337* alpha + 0.068991;

== matlab function Test_openloop/Dynamics in local/alpha calculation3 ==
  data: ptg input; psi output; theta output; gamma output
function [psi, theta, gamma] = fcn(ptg)
psi = ptg(1);
theta = ptg(2);
gamma = ptg(3);
end
